simulink model "Simulink_Control_BlueROVtest6"  (R2022b)
settings: Solver=VariableStepAuto  StartTime=0.0  StopTime=20  RelTol=1e-3
model workspace (MAT data in the model file):
  Minv = Simulink.Parameter
  Minv.Value = [0.0780640124902  0  0  0  0  0; 0  0.0499750124938  0  0  0  0; 0  0  0.0457038391225  0  0  0; 0  0  0  3.57142857143  0  0; 0  0  0  0  3.57142857143  0; 0  0  0  0  0  3.57142857143]
  Minv.DataType = 'auto'
  Minv.Complexity = 'real'
  Minv.Dimensions = [6 6]
values from neighbouring files (symbols this model uses):
  B = 0    [Control_BlueROV_Modo_Deslizante.m]
  C = 1    [Control_BlueROV_Modo_Deslizante.m]
  epsilong = 1    [Control_BlueROV_Modo_Deslizante.m]
  Ix = 0.1836    [Control_BlueROV_Modo_Deslizante.m]
  Ixy = 0    [Control_BlueROV_Modo_Deslizante.m]
  Ixz = 0    [Control_BlueROV_Modo_Deslizante.m]
  Iy = 0.2181    [Control_BlueROV_Modo_Deslizante.m]
  Iyz = -0.0021    [Control_BlueROV_Modo_Deslizante.m]
  Iz = 0.1482    [Control_BlueROV_Modo_Deslizante.m]
  K = 5    [Control_BlueROV_Modo_Deslizante.m]
  Kp = -5.005    [Control_BlueROV_Modo_Deslizante.m]
  Kpdot = -0.8576    [Control_BlueROV_Modo_Deslizante.m]
  Kpp = -80.25    [Control_BlueROV_Modo_Deslizante.m]
  m = 10.7668    [Control_BlueROV_Modo_Deslizante.m]
  M = Mrb+Ma    [Control_BlueROV_Modo_Deslizante.m]
  Minv = inv(M)    [Control_BlueROV_Modo_Deslizante.m]
  Mq = -5.005    [Control_BlueROV_Modo_Deslizante.m]
  Mqdot = -1.1214    [Control_BlueROV_Modo_Deslizante.m]
  Mqq = -80.25    [Control_BlueROV_Modo_Deslizante.m]
  Nr = -0.004    [Control_BlueROV_Modo_Deslizante.m]
  Nrdot = -0.7399    [Control_BlueROV_Modo_Deslizante.m]
  Nrr = -0.2506    [Control_BlueROV_Modo_Deslizante.m]
  W = 0    [Control_BlueROV_Modo_Deslizante.m]
  xb = 0    [Control_BlueROV_Modo_Deslizante.m]
  xg = 0    [Control_BlueROV_Modo_Deslizante.m]
  Xu = -0.0048    [Control_BlueROV_Modo_Deslizante.m]
  Xudot = -4.9063    [Control_BlueROV_Modo_Deslizante.m]
  Xuu = -30.61    [Control_BlueROV_Modo_Deslizante.m]
  yb = 0    [Control_BlueROV_Modo_Deslizante.m]
  yg = 0    [Control_BlueROV_Modo_Deslizante.m]
  Yv = -0.2437    [Control_BlueROV_Modo_Deslizante.m]
  Yvdot = -9.9210    (= -9.921)    [Control_BlueROV_Modo_Deslizante.m]
  Yvv = -38.0036    [Control_BlueROV_Modo_Deslizante.m]
  zb = 0.02    [Control_BlueROV_Modo_Deslizante.m]
  zg = 0    [Control_BlueROV_Modo_Deslizante.m]
  Zw = -0.0094    [Control_BlueROV_Modo_Deslizante.m]
  Zwdot = -17.6159    [Control_BlueROV_Modo_Deslizante.m]
  Zww = -62.5364    [Control_BlueROV_Modo_Deslizante.m]
libraries: simulink x1
(part 1 of 3)
settings Model: Creator=andres lopez  LastModifiedBy=Administrator
settings SolverCC: ZeroCrossAlgorithm=Adaptive  AlgebraicLoopSolver=TrustRegion
settings DebuggingCC: IgnoredZcDiagnostic=none  UnconnectedInputMsg=warning  UnconnectedOutputMsg=warning  UnconnectedLineMsg=warning  SFMachineParentedDataDiag=warning
settings ModelReferenceCC: EnableRefExpFcnMdlSchedulingChecks=on
settings SFSimCC: CustomCodeUndefinedFunction=UseInterfaceOnly

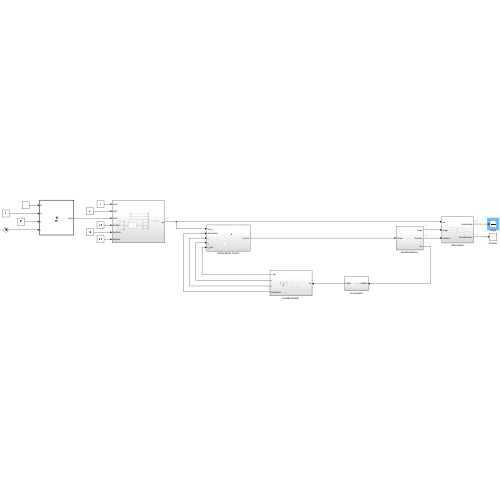
[thumbnail: Simulink's stored preview of the top-level diagram]
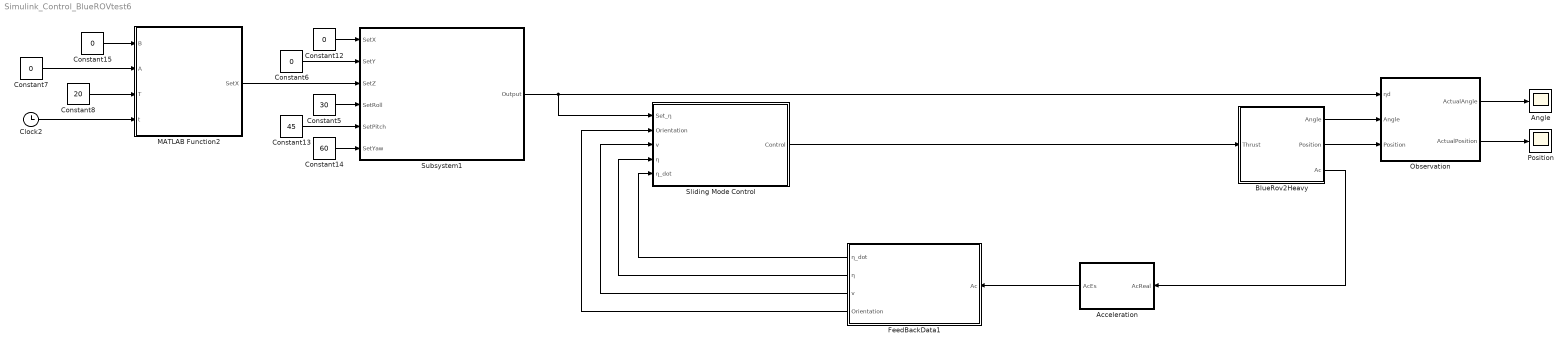
== system Simulink_Control_BlueROVtest6 ==
  Acceleration : Subsystem
  Angle : Scope
  BlueRov2Heavy : Subsystem
  Clock2 : Clock
  Constant{6..7,12,15} (4 alike) : Constant  Value=0
  Constant13 : Constant  Value=45
  Constant14 : Constant  Value=60
  Constant5 : Constant  Value=30
  Constant8 : Constant  Value=20
  FeedBackData1 : Subsystem
  MATLAB Function2 : MATLAB Function  TreatAsAtomicUnit=on
  Observation : Subsystem
  Position : Scope
  Sliding Mode Control : Subsystem
  Subsystem1 : Subsystem
  wires:
  Observation/1(ActualAngle) -> Angle/1
  BlueRov2Heavy/1(Angle) -> Observation/2(Angle)
  Observation/2(ActualPosition) -> Position/1
  Constant14/1 -> Subsystem1/6(SetYaw)
  Constant6/1 -> Subsystem1/2(SetY)
  Constant8/1 -> MATLAB Function2/3(T)
  Clock2/1 -> MATLAB Function2/4(t)
  Constant13/1 -> Subsystem1/5(SetPitch)
  Constant15/1 -> MATLAB Function2/1(B)
  Constant5/1 -> Subsystem1/4(SetRoll)
  Constant7/1 -> MATLAB Function2/2(A)
  Constant12/1 -> Subsystem1/1(SetX)
  MATLAB Function2/1(SetX) -> Subsystem1/3(SetZ)
  BlueRov2Heavy/2(Position) -> Observation/3(Position)
  Acceleration/1(AcEs) -> FeedBackData1/1(Ac)
  BlueRov2Heavy/3(Ac) -> Acceleration/1(AcReal)
  FeedBackData1/1(η_dot) -> Sliding Mode Control/5(η_dot)
  FeedBackData1/2(η) -> Sliding Mode Control/4(η)
  FeedBackData1/3(v) -> Sliding Mode Control/3(v)
  FeedBackData1/4(Orientation) -> Sliding Mode Control/2(Orientation)
  Subsystem1/1(Output) -> Observation/1(ηd), Sliding Mode Control/1(Set_η)
  Sliding Mode Control/1(Control) -> BlueRov2Heavy/1(Thrust)

== system Simulink_Control_BlueROVtest6/Acceleration ==
  AcReal : Inport
  Gain : Gain
  AcEs : Outport  VectorParamsAs1DForOutWhenUnconnected=off
  wires:
  Gain/1 -> AcEs/1
  AcReal/1 -> Gain/1

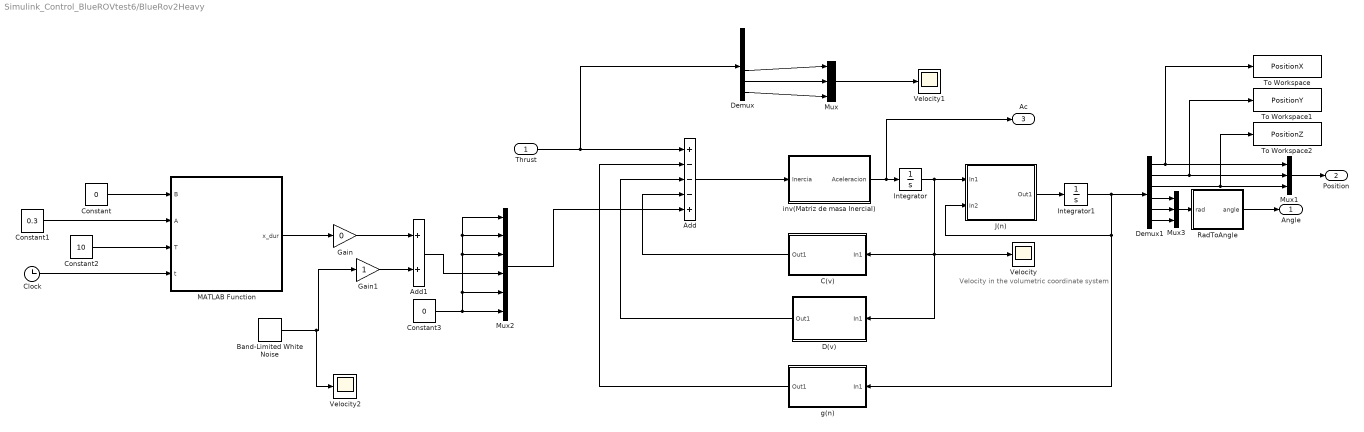
== system Simulink_Control_BlueROVtest6/BlueRov2Heavy ==
  note: Velocity in the volumetric coordinate system
  Thrust : Inport
  Add : Sum  Inputs=+---+
  Add1 : Sum
  Band-Limited White Noise : simulink/Sources/Band-Limited White Noise  Cov=[0.1]  Ts=0.1  seed=[23341]
  C(v) : Subsystem
  Clock : Clock
  Constant : Constant  Value=0
  Constant1 : Constant  Value=0.3
  Constant2 : Constant  Value=10
  Constant3 : Constant  Value=0
  D(v) : Subsystem
  Demux : Demux  Outputs=6
  Demux1 : Demux  Outputs=6
  Gain : Gain  Gain=0
  Gain1 : Gain
  Integrator : Integrator
  Integrator1 : Integrator
  J(n) : Subsystem
  MATLAB Function : MATLAB Function  TreatAsAtomicUnit=on
  Mux : Mux  Inputs=3
  Mux1 : Mux  Inputs=3
  Mux2 : Mux  Inputs=6
  Mux3 : Mux  Inputs=3
  RadToAngle : Subsystem
  To Workspace : ToWorkspace  VariableName=PositionX  SampleTime=-1
  To Workspace1 : ToWorkspace  VariableName=PositionY  SampleTime=-1
  To Workspace2 : ToWorkspace  VariableName=PositionZ  SampleTime=-1
  Velocity : Scope
  Velocity1 : Scope
  Velocity2 : Scope
  g(n) : Subsystem
  inv(Matriz de masa Inercial) : Subsystem
  Angle : Outport  VectorParamsAs1DForOutWhenUnconnected=off
  Position : Outport  Port=2  VectorParamsAs1DForOutWhenUnconnected=off
  Ac : Outport  Port=3  VectorParamsAs1DForOutWhenUnconnected=off
  wires:
  Thrust/1 -> Demux/1, Add/1
  Add/1 -> inv(Matriz de masa Inercial)/1(Inercia)
  J(n)/1(Out1) -> Integrator1/1
  inv(Matriz de masa Inercial)/1(Aceleracion) -> Ac/1, Integrator/1
  g(n)/1(Out1) -> Add/2
  Integrator1/1 -> g(n)/1(In1), J(n)/2(In2), Demux1/1
  Integrator/1 -> Velocity/1, D(v)/1(In1), C(v)/1(In1), J(n)/1(In1)
  C(v)/1(Out1) -> Add/4
  Demux1/2 -> To Workspace1/1, Mux1/2
  Demux1/3 -> To Workspace2/1, Mux1/3
  Demux1/1 -> To Workspace/1, Mux1/1
  Mux1/1 -> Position/1
  D(v)/1(Out1) -> Add/3
  Constant/1 -> MATLAB Function/1(B)
  Constant1/1 -> MATLAB Function/2(A)
  Constant2/1 -> MATLAB Function/3(T)
  Clock/1 -> MATLAB Function/4(t)
  Mux2/1 -> Add/5
  Constant3/1 -> Mux2/3, Mux2/2, Mux2/1, Mux2/5, Mux2/6
  MATLAB Function/1(x_dur) -> Gain/1
  Gain/1 -> Add1/1
  Gain1/1 -> Add1/2
  Mux3/1 -> RadToAngle/1(rad)
  Demux1/5 -> Mux3/2
  Demux1/4 -> Mux3/1
  Demux1/6 -> Mux3/3
  RadToAngle/1(angle) -> Angle/1
  Band-Limited White Noise/1 -> Velocity2/1, Gain1/1
  Demux/4 -> Mux/1
  Demux/5 -> Mux/2
  Demux/6 -> Mux/3
  Mux/1 -> Velocity1/1
  Add1/1 -> Mux2/4

== system Simulink_Control_BlueROVtest6/FeedBackData1 ==
  note: 输入：体坐标系中的线加速度与角加速度
  note: 输出1：世界坐标系中的位置与角度
  note: 输出4：世界坐标系中的机器人角度信息
  Ac : Inport
  Demux : Demux  Outputs=6
  Demux1 : Demux  Outputs=3
  Integrator : Integrator
  Integrator1 : Integrator
  J(n) : Subsystem
  Mux : Mux  Inputs=6
  Mux1 : Mux  Inputs=3
  η_dot : Outport
  η : Outport  Port=2  VectorParamsAs1DForOutWhenUnconnected=off
  v : Outport  Port=3
  Orientation : Outport  Port=4  VectorParamsAs1DForOutWhenUnconnected=off
  wires:
  Ac/1 -> Integrator/1
  Integrator/1 -> v/1, J(n)/1(In1)
  J(n)/1(Output) -> η_dot/1, Integrator1/1
  Integrator1/1 -> Demux/1
  Demux/1 -> Mux/1
  Demux/2 -> Mux/2
  Demux1/2 -> Mux/5
  Demux1/1 -> Mux/4
  Demux1/3 -> Mux/6
  Mux/1 -> η/1
  Demux/3 -> Mux/3
  Mux1/1 -> Orientation/1, J(n)/2(In2), Demux1/1
  Demux/4 -> Mux1/1
  Demux/5 -> Mux1/2
  Demux/6 -> Mux1/3

== system Simulink_Control_BlueROVtest6/Observation ==
  ηd : Inport
  Angle : Inport  Port=2
  Position : Inport  Port=3
  Demux : Demux  Outputs=2
  Mux : Mux  Inputs=2
  Mux1 : Mux  Inputs=2
  RadToAngle : Subsystem
  ActualAngle : Outport
  ActualPosition : Outport  Port=2
  wires:
  Demux/1 -> Mux/1
  Position/1 -> Mux/2
  Demux/2 -> RadToAngle/1(rad)
  Mux1/1 -> ActualAngle/1
  Mux/1 -> ActualPosition/1
  ηd/1 -> Demux/1
  RadToAngle/1(angle) -> Mux1/1
  Angle/1 -> Mux1/2

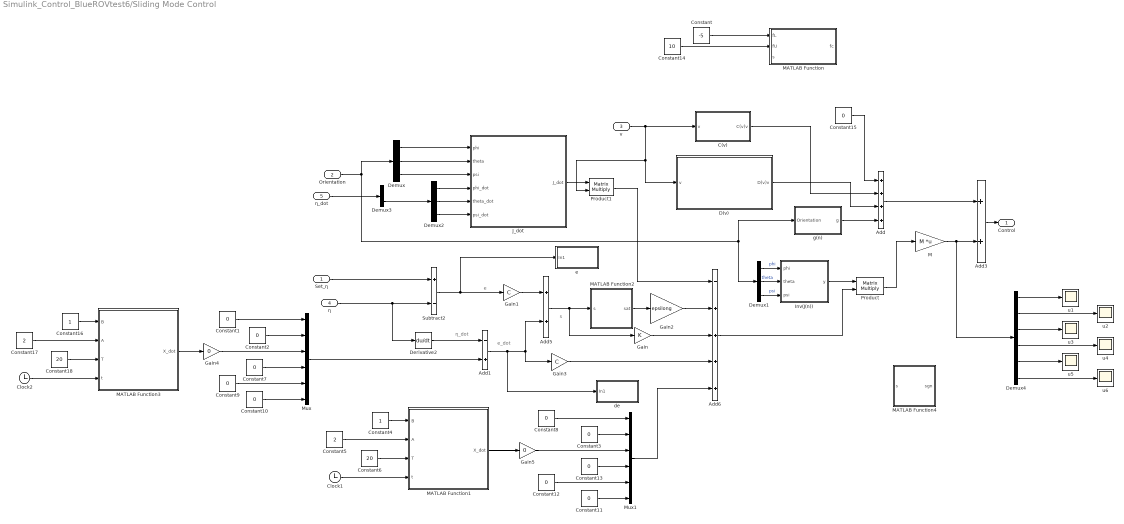
== system Simulink_Control_BlueROVtest6/Sliding Mode Control ==
  note: η_dot
  note: s
  note: e
  note: e_dot
  Set_η : Inport
  Orientation : Inport  Port=2
  v : Inport  Port=3
  η : Inport  Port=4
  η_dot : Inport  Port=5
  Add : Sum  Inputs=++++
  Add1 : Sum  Inputs=-+
  Add3 : Sum
  Add5 : Sum
  Add6 : Sum  Inputs=-++++
  C(v) : Subsystem
  Clock1 : Clock
  Clock2 : Clock
  Constant : Constant  Value=-5
  Constant{1..3,7..13,15} (11 alike) : Constant  Value=0
  Constant14 : Constant  Value=10
  Constant16 : Constant
  Constant17 : Constant  Value=2
  Constant18 : Constant  Value=20
  Constant4 : Constant
  Constant5 : Constant  Value=2
  Constant6 : Constant  Value=20
  D(v) : Subsystem
  Demux : Demux  Outputs=3
  Demux1 : Demux  Outputs=3
  Demux2 : Demux  Outputs=3
  Demux3 : Demux  Outputs=2
  Demux4 : Demux  Outputs=6
  Derivative2 : Derivative
  Gain : Gain  Gain=K
  Gain1 : Gain  Gain=C
  Gain2 : Gain  Gain=epsilong
  Gain3 : Gain  Gain=C
  Gain4 : Gain  Gain=0
  Gain5 : Gain  Gain=0
  Inv(J(n)) : MATLAB Function  TreatAsAtomicUnit=on
  J_dot : MATLAB Function  TreatAsAtomicUnit=on
  M : Gain  Gain=M  Multiplication=Matrix(K*u) (u vector)
  MATLAB Function : MATLAB Function  TreatAsAtomicUnit=on
  MATLAB Function1 : MATLAB Function  TreatAsAtomicUnit=on
  MATLAB Function2 : MATLAB Function  TreatAsAtomicUnit=on
  MATLAB Function3 : MATLAB Function  TreatAsAtomicUnit=on
  MATLAB Function4 : MATLAB Function  TreatAsAtomicUnit=on
  Mux : Mux  Inputs=6
  Mux1 : Mux  Inputs=6
  Product : Product  Multiplication=Matrix(*)
  Product1 : Product  Multiplication=Matrix(*)
  Subtract2 : Sum  Inputs=+-
  de : Subsystem
  e : Subsystem
  g(n) : Subsystem
  u{1..6} (6 alike) : Scope
  Control : Outport  VectorParamsAs1DForOutWhenUnconnected=off
  wires:
  Orientation/1 -> g(n)/1(Orientation), Demux1/1, Demux/1
  Demux1/1 -> Inv(J(n))/1(phi)  "phi"
  Demux1/3 -> Inv(J(n))/3(psi)  "psi"
  Inv(J(n))/1(y) -> Product/1
  Demux1/2 -> Inv(J(n))/2(theta)  "theta"
  Add3/1 -> Control/1
  M/1 -> Add3/2, Demux4/1
  Add/1 -> Add3/1
  η/1 -> Derivative2/1, Subtract2/2
  Set_η/1 -> Subtract2/1
  v/1 -> D(v)/1(v), Product1/2, C(v)/1(v)
  Add1/1 -> de/1(In1), Add5/2, Gain3/1
  Gain1/1 -> Add5/1
  Add5/1 -> MATLAB Function2/1(s), Gain/1
  Add6/1 -> Product/2
  Subtract2/1 -> e/1(In1), Gain1/1
  Product/1 -> M/1
  Demux/1 -> J_dot/1(phi)
  Demux/2 -> J_dot/2(theta)
  Demux/3 -> J_dot/3(psi)
  Demux2/1 -> J_dot/4(phi_dot)
  Demux2/2 -> J_dot/5(theta_dot)
  Demux2/3 -> J_dot/6(psi_dot)
  Gain/1 -> Add6/3
  Product1/1 -> Add6/1
  J_dot/1(J_dot) -> Product1/1
  Gain3/1 -> Add6/4
  Demux3/2 -> Demux2/1
  η_dot/1 -> Demux3/1
  Derivative2/1 -> Add1/1
  Constant7/1 -> Mux/4
  Constant10/1 -> Mux/6
  Constant9/1 -> Mux/5
  Constant11/1 -> Mux1/6
  Constant12/1 -> Mux1/5
  Constant13/1 -> Mux1/4
  Mux/1 -> Add1/2
  Mux1/1 -> Add6/5
  Constant18/1 -> MATLAB Function3/3(T)
  Constant16/1 -> MATLAB Function3/1(B)
  Constant17/1 -> MATLAB Function3/2(A)
  Clock2/1 -> MATLAB Function3/4(t)
  MATLAB Function1/1(X_dot) -> Gain5/1
  Gain2/1 -> Add6/2
  MATLAB Function2/1(sat) -> Gain2/1
  MATLAB Function3/1(X_dot) -> Gain4/1
  Constant2/1 -> Mux/2
  Constant3/1 -> Mux1/2
  Constant4/1 -> MATLAB Function1/1(B)
  Constant5/1 -> MATLAB Function1/2(A)
  Clock1/1 -> MATLAB Function1/4(t)
  Constant6/1 -> MATLAB Function1/3(T)
  Constant1/1 -> Mux/1
  Constant8/1 -> Mux1/1
  Demux4/1 -> u1/1
  Demux4/2 -> u2/1
  Demux4/3 -> u3/1
  Demux4/4 -> u4/1
  Demux4/5 -> u5/1
  Demux4/6 -> u6/1
  Constant14/1 -> MATLAB Function/2(fU)
  Constant/1 -> MATLAB Function/1(fL)
  g(n)/1(g) -> Add/4
  D(v)/1(D(v)v) -> Add/3
  C(v)/1(C(v)v) -> Add/2
  Constant15/1 -> Add/1
  Gain4/1 -> Mux/3
  Gain5/1 -> Mux1/3

== system Simulink_Control_BlueROVtest6/Subsystem1 ==
  SetX : Inport
  SetY : Inport  Port=2
  SetZ : Inport  Port=3
  SetRoll : Inport  Port=4
  SetPitch : Inport  Port=5
  SetYaw : Inport  Port=6
  AngleToRad : Subsystem
  Demux : Demux  Outputs=3
  Mux : Mux  Inputs=3
  Mux1 : Mux  Inputs=6
  Output : Outport
  wires:
  SetY/1 -> Mux1/2
  Mux1/1 -> Output/1  "ηd"
  SetZ/1 -> Mux1/3
  SetX/1 -> Mux1/1
  Demux/1 -> Mux1/4
  Demux/2 -> Mux1/5
  Demux/3 -> Mux1/6
  AngleToRad/1(Rad) -> Demux/1
  Mux/1 -> AngleToRad/1(Angle)
  SetRoll/1 -> Mux/1
  SetPitch/1 -> Mux/2
  SetYaw/1 -> Mux/3

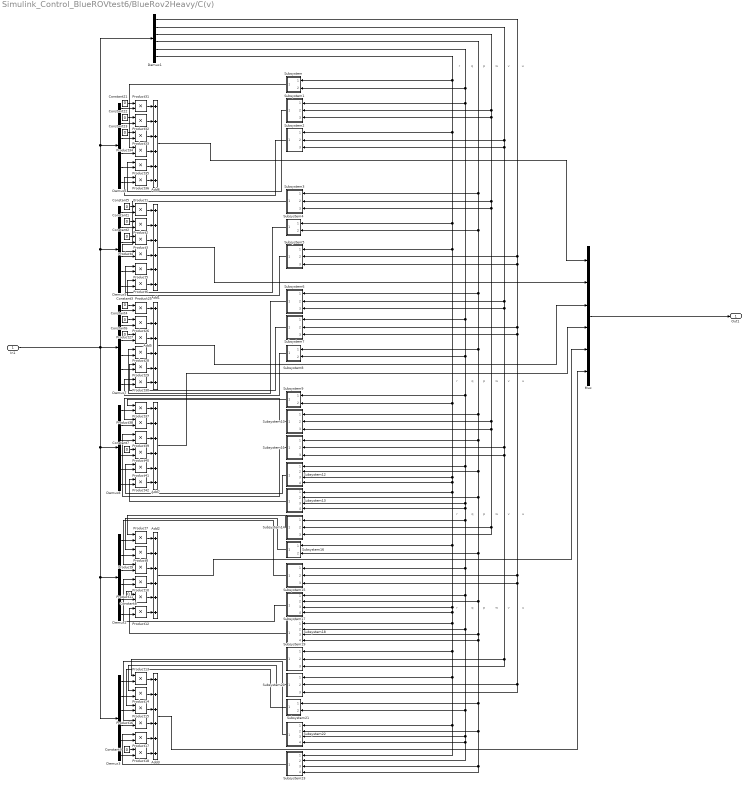
== system Simulink_Control_BlueROVtest6/BlueRov2Heavy/C(v) ==
  note: u
  note: v
  note: w
  note: p
  note: q
  note: r
  note: v
  note: p
  note: u
  note: w
  note: q
  note: r
  note: v
  note: r
  note: w
  note: u
  note: q
  note: p
  note: v
  note: r
  note: w
  note: u
  note: q
  note: p
  In1 : Inport
  Add{1..3,5..7} (6 alike) : Sum  Inputs=++++++
  Constant{1..9,21..23} (12 alike) : Constant  Value=0
  Demux{1..3,5..8} (7 alike) : Demux  Outputs=6
  Mux : Mux  Inputs=6
  Product{1..18,25..42} (36 alike) : Product
  Subsystem : Subsystem
  Subsystem1 : Subsystem
  Subsystem10 : Subsystem
  Subsystem11 : Subsystem
  Subsystem12 : Subsystem
  Subsystem13 : Subsystem
  Subsystem14 : Subsystem
  Subsystem15 : Subsystem
  Subsystem16 : Subsystem
  Subsystem17 : Subsystem
  Subsystem18 : Subsystem
  Subsystem19 : Subsystem
  Subsystem2 : Subsystem
  Subsystem20 : Subsystem
  Subsystem21 : Subsystem
  Subsystem22 : Subsystem
  Subsystem23 : Subsystem
  Subsystem3 : Subsystem
  Subsystem4 : Subsystem
  Subsystem5 : Subsystem
  Subsystem6 : Subsystem
  Subsystem7 : Subsystem
  Subsystem8 : Subsystem
  Subsystem9 : Subsystem
  Out1 : Outport  VectorParamsAs1DForOutWhenUnconnected=off
  wires:
  In1/1 -> Demux5/1, Demux6/1, Demux1/1, Demux7/1, Demux8/1, Demux3/1, Demux2/1
  Product39/1 -> Add7/3
  Demux8/2 -> Product38/2
  Product36/1 -> Add6/6
  Product31/1 -> Add6/1
  Product35/1 -> Add6/5
  Demux6/2 -> Product32/2
  Demux6/4 -> Product34/2
  Demux6/5 -> Product35/2
  Product33/1 -> Add6/3
  Demux6/3 -> Product33/2
  Product5/1 -> Add1/5
  Demux5/2 -> Product2/2
  Product32/1 -> Add6/2
  Product41/1 -> Add7/5
  Product34/1 -> Add6/4
  Product2/1 -> Add1/2
  Demux8/5 -> Product41/2
  Product1/1 -> Add1/1
  Product18/1 -> Add3/6
  Product3/1 -> Add1/3
  Demux8/3 -> Product39/2
  Product8/1 -> Add2/2
  Demux2/6 -> Product12/2
  Product4/1 -> Add1/4
  Product37/1 -> Add7/1
  Demux5/1 -> Product1/2
  Demux8/6 -> Product42/2
  Demux5/4 -> Product4/2
  Demux5/5 -> Product5/2
  Product17/1 -> Add3/5
  Demux5/3 -> Product3/2
  Demux6/1 -> Product31/2
  Product13/1 -> Add3/1
  Product14/1 -> Add3/2
  Product40/1 -> Add7/4
  Product15/1 -> Add3/3
  Demux8/4 -> Product40/2
  Demux7/2 -> Product26/2
  Product42/1 -> Add7/6
  Product12/1 -> Add2/6
  Product26/1 -> Add5/2
  Product6/1 -> Add1/6
  Demux6/6 -> Product36/2
  Demux5/6 -> Product6/2
  Product29/1 -> Add5/5
  Product28/1 -> Add5/4
  Demux7/3 -> Product27/2
  Product16/1 -> Add3/4
  Product10/1 -> Add2/4
  Demux7/5 -> Product29/2
  Product9/1 -> Add2/3
  Product38/1 -> Add7/2
  Demux2/4 -> Product10/2
  Demux2/2 -> Product8/2
  Demux8/1 -> Product37/2
  Demux2/5 -> Product11/2
  Product7/1 -> Add2/1
  Product11/1 -> Add2/5
  Mux/1 -> Out1/1
  Demux7/4 -> Product28/2
  Demux2/1 -> Product7/2
  Demux7/6 -> Product30/2
  Product25/1 -> Add5/1
  Product27/1 -> Add5/3
  Product30/1 -> Add5/6
  Demux7/1 -> Product25/2
  Demux2/3 -> Product9/2
  Constant21/1 -> Product31/1
  Constant22/1 -> Product32/1
  Constant23/1 -> Product33/1
  Demux3/6 -> Product18/2
  Demux3/5 -> Product17/2
  Demux3/4 -> Product16/2
  Demux3/3 -> Product15/2
  Demux3/2 -> Product14/2
  Demux3/1 -> Product13/2
  Constant5/1 -> Product1/1
  Constant1/1 -> Product2/1
  Constant2/1 -> Product3/1
  Constant3/1 -> Product25/1
  Constant4/1 -> Product26/1
  Constant6/1 -> Product27/1
  Constant7/1 -> Product40/1
  Constant8/1 -> Product11/1
  Constant9/1 -> Product18/1
  Demux1/1 -> Subsystem5/2(In2), Subsystem15/2(In2), Subsystem15/3(In3), Subsystem20/2(In2), Subsystem20/3(In3), Subsystem7/3(In3), Subsystem7/2(In2), Subsystem5/3(In3)
  Demux1/2 -> Subsystem11/3(In3), Subsystem19/2(In2), Subsystem19/3(In3), Subsystem11/2(In2), Subsystem6/3(In3), Subsystem6/2(In2), Subsystem2/3(In3), Subsystem2/2(In2)
  Demux1/3 -> Subsystem3/2(In2), Subsystem3/3(In3), Subsystem10/2(In2), Subsystem10/3(In3), Subsystem14/2(In2), Subsystem14/3(In3), Subsystem1/3(In3), Subsystem1/2(In2)
  Subsystem/1(Out1) -> Product34/1
  Subsystem1/1(Out1) -> Product35/1
  Subsystem2/1(Out1) -> Product36/1
  Add6/1 -> Mux/1
  Subsystem3/1(Out1) -> Product4/1
  Subsystem4/1(Out1) -> Product5/1
  Subsystem5/1(Out1) -> Product6/1
  Add1/1 -> Mux/2
  Subsystem6/1(Out1) -> Product28/1
  Subsystem7/1(Out1) -> Product29/1
  Subsystem8/1(Out1) -> Product30/1
  Add5/1 -> Mux/3
  Subsystem9/1(Out1) -> Product37/1
  Subsystem10/1(Out1) -> Product38/1
  Subsystem11/1(Out1) -> Product39/1
  Subsystem12/1(Out1) -> Product41/1
  Subsystem13/1(Out1) -> Product42/1
  Add7/1 -> Mux/4
  Subsystem14/1(Out1) -> Product7/1
  Demux1/4 -> Subsystem3/1(In1), Subsystem4/2(In2), Subsystem8/1(In1), Subsystem10/1(In1), Subsystem11/1(In1), Subsystem12/2(In2), Subsystem13/2(In2), Subsystem16/2(In2), Subsystem17/2(In2), Subsystem18/3(In3), Subsystem18/4(In4), Subsystem21/1(In1), Subsystem22/2(In2), Subsystem23/3(In3), Subsystem23/4(In4), Subsystem6/1(In1)
  Subsystem16/1(Out1) -> Product8/1
  Subsystem15/1(Out1) -> Product9/1
  Demux1/6 -> Subsystem4/1(In1), Subsystem5/1(In1), Subsystem12/4(In4), Subsystem13/1(In1), Subsystem16/1(In1), Subsystem17/4(In4), Subsystem18/1(In1), Subsystem19/1(In1), Subsystem20/1(In1), Subsystem22/1(In1), Subsystem23/1(In1), Subsystem17/3(In3), Subsystem12/3(In3), Subsystem9/2(In2), Subsystem2/1(In1), Subsystem/1(In1)
  Subsystem17/1(Out1) -> Product10/1
  Subsystem18/1(Out1) -> Product12/1
  Subsystem19/1(Out1) -> Product13/1
  Add2/1 -> Mux/5
  Subsystem20/1(Out1) -> Product14/1
  Subsystem21/1(Out1) -> Product15/1
  Demux1/5 -> Subsystem12/1(In1), Subsystem13/3(In3), Subsystem13/4(In4), Subsystem15/1(In1), Subsystem17/1(In1), Subsystem18/2(In2), Subsystem21/2(In2), Subsystem22/4(In4), Subsystem23/2(In2), Subsystem22/3(In3), Subsystem14/1(In1), Subsystem9/1(In1), Subsystem8/2(In2), Subsystem7/1(In1), Subsystem1/1(In1), Subsystem/2(In2)
  Subsystem22/1(Out1) -> Product16/1
  Subsystem23/1(Out1) -> Product17/1
  Add3/1 -> Mux/6

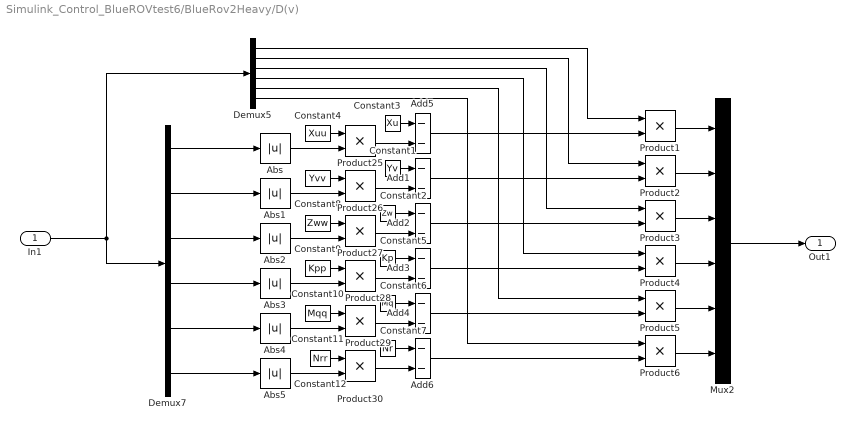
== system Simulink_Control_BlueROVtest6/BlueRov2Heavy/D(v) ==
  In1 : Inport
  Abs{,1..5} (6 alike) : Abs  SaturateOnIntegerOverflow=off
  Add{1..6} (6 alike) : Sum  Inputs=--
  Constant1 : Constant  Value=Yv
  Constant10 : Constant  Value=Kpp
  Constant11 : Constant  Value=Mqq
  Constant12 : Constant  Value=Nrr
  Constant2 : Constant  Value=Zw
  Constant3 : Constant  Value=Xu
  Constant4 : Constant  Value=Xuu
  Constant5 : Constant  Value=Kp
  Constant6 : Constant  Value=Mq
  Constant7 : Constant  Value=Nr
  Constant8 : Constant  Value=Yvv
  Constant9 : Constant  Value=Zww
  Demux5 : Demux  Outputs=6
  Demux7 : Demux  Outputs=6
  Mux2 : Mux  Inputs=6
  Product{1..6,25..30} (12 alike) : Product
  Out1 : Outport
  wires:
  Demux5/5 -> Product5/1
  Demux7/3 -> Abs2/1
  Abs/1 -> Product25/2
  Demux7/5 -> Abs4/1
  Constant9/1 -> Product27/1
  Constant6/1 -> Add4/1
  Mux2/1 -> Out1/1
  Constant1/1 -> Add1/1
  Product5/1 -> Mux2/5
  Abs1/1 -> Product26/2
  Product4/1 -> Mux2/4
  Constant2/1 -> Add2/1
  Demux7/4 -> Abs3/1
  Demux7/6 -> Abs5/1
  Constant12/1 -> Product30/1
  In1/1 -> Demux5/1, Demux7/1
  Product1/1 -> Mux2/1
  Demux7/1 -> Abs/1
  Product29/1 -> Add4/2
  Add3/1 -> Product4/2
  Constant10/1 -> Product28/1
  Add1/1 -> Product2/2
  Demux7/2 -> Abs1/1
  Product26/1 -> Add1/2
  Demux5/2 -> Product2/1
  Add4/1 -> Product5/2
  Demux5/4 -> Product4/1
  Abs5/1 -> Product30/2
  Product3/1 -> Mux2/3
  Product6/1 -> Mux2/6
  Abs3/1 -> Product28/2
  Constant4/1 -> Product25/1
  Constant11/1 -> Product29/1
  Product28/1 -> Add3/2
  Product25/1 -> Add5/2
  Abs2/1 -> Product27/2
  Constant7/1 -> Add6/1
  Demux5/6 -> Product6/1
  Product27/1 -> Add2/2
  Add2/1 -> Product3/2
  Constant3/1 -> Add5/1
  Product30/1 -> Add6/2
  Abs4/1 -> Product29/2
  Constant5/1 -> Add3/1
  Product2/1 -> Mux2/2
  Demux5/1 -> Product1/1
  Constant8/1 -> Product26/1
  Add5/1 -> Product1/2
  Demux5/3 -> Product3/1
  Add6/1 -> Product6/2

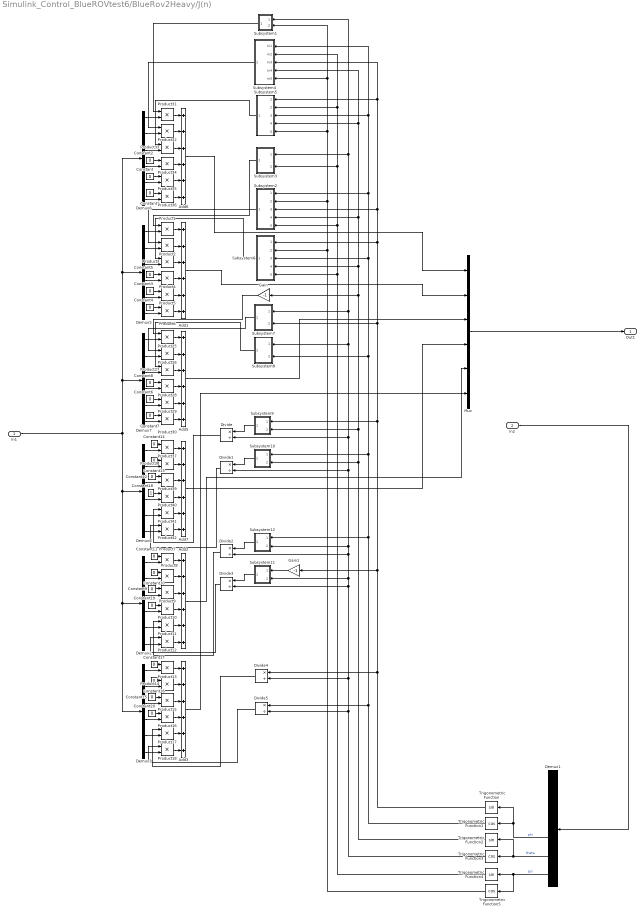
== system Simulink_Control_BlueROVtest6/BlueRov2Heavy/J(n) ==
  In1 : Inport
  In2 : Inport  Port=2
  Add{1..3,5..7} (6 alike) : Sum  Inputs=++++++
  Constant{,1..17,19..20} (20 alike) : Constant  Value=0
  Constant18 : Constant
  Demux{1..3,5..8} (7 alike) : Demux  Outputs=6
  Divide{,1..5} (6 alike) : Product  Inputs=*/
  Gain : Gain  Gain=-1
  Gain1 : Gain  Gain=-1
  Mux : Mux  Inputs=6
  Product{1..18,25..42} (36 alike) : Product
  Subsystem1 : Subsystem
  Subsystem10 : Subsystem
  Subsystem11 : Subsystem
  Subsystem12 : Subsystem
  Subsystem2 : Subsystem
  Subsystem3 : Subsystem
  Subsystem4 : Subsystem
  Subsystem5 : Subsystem
  Subsystem6 : Subsystem
  Subsystem7 : Subsystem
  Subsystem8 : Subsystem
  Subsystem9 : Subsystem
  Trigonometric Function : Trigonometry
  Trigonometric Function1 : Trigonometry  Operator=cos
  Trigonometric Function2 : Trigonometry
  Trigonometric Function3 : Trigonometry  Operator=cos
  Trigonometric Function4 : Trigonometry
  Trigonometric Function5 : Trigonometry  Operator=cos
  Out1 : Outport  VectorParamsAs1DForOutWhenUnconnected=off
  wires:
  Divide5/1 -> Product18/1
  Divide3/1 -> Product12/1
  Subsystem1/1(Out1) -> Product31/1
  Constant12/1 -> Product39/1
  Subsystem5/1(Out1) -> Product33/1
  Constant13/1 -> Product38/1
  Subsystem10/1(Out1) -> Divide1/1
  Divide1/1 -> Product42/1
  Demux7/3 -> Product27/2
  Product28/1 -> Add5/4
  Product29/1 -> Add5/5
  Product25/1 -> Add5/1
  Product30/1 -> Add5/6
  Demux7/6 -> Product30/2
  Constant8/1 -> Product28/1
  Demux7/1 -> Product25/2
  Demux7/4 -> Product28/2
  Product27/1 -> Add5/3
  Constant6/1 -> Product29/1
  Product11/1 -> Add2/5
  Demux2/3 -> Product9/2
  Product7/1 -> Add2/1
  Demux2/1 -> Product7/2
  Demux2/5 -> Product11/2
  Demux2/4 -> Product10/2
  Product9/1 -> Add2/3
  Demux2/2 -> Product8/2
  Constant10/1 -> Product8/1
  Trigonometric Function3/1 -> Divide5/2, Divide4/2, Divide3/2, Subsystem11/2(In2), Divide2/2, Subsystem12/2(In2), Divide1/2, Divide/2, Subsystem8/1(In1), Subsystem7/1(In1), Subsystem3/1(In1), Subsystem1/1(In1)
  Demux8/2 -> Product38/2
  Product39/1 -> Add7/3
  Product38/1 -> Add7/2
  In1/1 -> Demux5/1, Demux6/1, Demux7/1, Demux8/1, Demux3/1, Demux2/1
  Subsystem9/1(Out1) -> Divide/1
  Add2/1 -> Mux/5
  Subsystem11/1(Out1) -> Divide3/1
  Product10/1 -> Add2/4
  Subsystem12/1(Out1) -> Divide2/1
  Constant19/1 -> Product10/1
  Trigonometric Function1/1 -> Divide5/1, Subsystem10/1(In1), Subsystem8/2(In2), Subsystem6/3(In3), Subsystem2/1(In1), Subsystem5/3(In3), Subsystem4/1(In1), Subsystem12/1(In1)
  Add1/1 -> Mux/2
  Mux/1 -> Out1/1
  Add6/1 -> Mux/1
  Add3/1 -> Mux/6
  Product12/1 -> Add2/6
  Add7/1 -> Mux/4
  Divide4/1 -> Product17/1
  Add5/1 -> Mux/3
  Product26/1 -> Add5/2
  Constant7/1 -> Product30/1
  Trigonometric Function/1 -> Divide4/1, Gain1/1, Subsystem9/1(In1), Subsystem7/2(In2), Subsystem6/1(In1), Subsystem2/3(In3), Subsystem5/1(In1), Subsystem4/3(In3)
  Constant14/1 -> Product37/1
  Gain/1 -> Product25/1
  Trigonometric Function5/1 -> Subsystem6/2(In2), Subsystem5/5(In5), Subsystem4/5(In5), Subsystem1/2(In2), Subsystem2/2(In2)
  Subsystem8/1(Out1) -> Product27/1
  Subsystem3/1(Out1) -> Product1/1
  Subsystem6/1(Out1) -> Product3/1
  Demux7/2 -> Product26/2
  Constant20/1 -> Product16/1
  Subsystem7/1(Out1) -> Product26/1
  Demux7/5 -> Product29/2
  Constant15/1 -> Product15/1
  Constant16/1 -> Product14/1
  Demux3/2 -> Product14/2
  Product15/1 -> Add3/3
  Constant17/1 -> Product13/1
  Product14/1 -> Add3/2
  Constant11/1 -> Product7/1
  Trigonometric Function4/1 -> Subsystem6/5(In5), Subsystem2/5(In5), Subsystem3/2(In2), Subsystem5/2(In2), Subsystem4/2(In2)
  Subsystem4/1(Out1) -> Product32/1
  Product13/1 -> Add3/1
  Product16/1 -> Add3/4
  Demux3/1 -> Product13/2
  Demux3/4 -> Product16/2
  Demux3/3 -> Product15/2
  Trigonometric Function2/1 -> Subsystem10/2(In2), Subsystem9/2(In2), Gain/1, Subsystem6/4(In4), Subsystem2/4(In4), Subsystem5/4(In4), Subsystem4/4(In4)
  Constant1/1 -> Product36/1
  Product17/1 -> Add3/5
  Demux5/3 -> Product3/2
  Product6/1 -> Add1/6
  Demux5/5 -> Product5/2
  Demux5/4 -> Product4/2
  Demux5/1 -> Product1/2
  Demux1/4 -> Trigonometric Function/1, Trigonometric Function1/1  "phi"
  Constant4/1 -> Product6/1
  Constant2/1 -> Product34/1
  Constant/1 -> Product35/1
  Demux8/6 -> Product42/2
  Demux3/5 -> Product17/2
  Product4/1 -> Add1/4
  Constant18/1 -> Product40/1
  Product37/1 -> Add7/1
  Demux2/6 -> Product12/2
  Demux8/4 -> Product40/2
  Gain1/1 -> Subsystem11/1(In1)
  Product42/1 -> Add7/6
  Constant3/1 -> Product5/1
  Product8/1 -> Add2/2
  Demux8/5 -> Product41/2
  Product1/1 -> Add1/1
  Demux8/3 -> Product39/2
  Product3/1 -> Add1/3
  Divide2/1 -> Product11/1
  Product18/1 -> Add3/6
  Demux1/6 -> Trigonometric Function5/1, Trigonometric Function4/1  "psi"
  Constant5/1 -> Product4/1
  Demux5/2 -> Product2/2
  Divide/1 -> Product41/1
  Product32/1 -> Add6/2
  Product2/1 -> Add1/2
  Product34/1 -> Add6/4
  Demux6/1 -> Product31/2
  Demux6/6 -> Product36/2
  Product41/1 -> Add7/5
  Demux6/5 -> Product35/2
  Product5/1 -> Add1/5
  Constant9/1 -> Product9/1
  Demux3/6 -> Product18/2
  Product33/1 -> Add6/3
  Demux1/5 -> Trigonometric Function2/1, Trigonometric Function3/1  "theta"
  Demux6/4 -> Product34/2
  Demux6/3 -> Product33/2
  Demux5/6 -> Product6/2
  Product36/1 -> Add6/6
  Demux6/2 -> Product32/2
  Subsystem2/1(Out1) -> Product2/1
  Product40/1 -> Add7/4
  Demux8/1 -> Product37/2
  Product31/1 -> Add6/1
  Product35/1 -> Add6/5
  In2/1 -> Demux1/1

== system Simulink_Control_BlueROVtest6/BlueRov2Heavy/RadToAngle ==
  rad : Inport
  Constant6 : Constant  Value=180
  Constant7 : Constant  Value=3.141592657
  Divide1 : Product  Inputs=*/*
  angle : Outport
  wires:
  Constant6/1 -> Divide1/3
  rad/1 -> Divide1/1
  Divide1/1 -> angle/1
  Constant7/1 -> Divide1/2

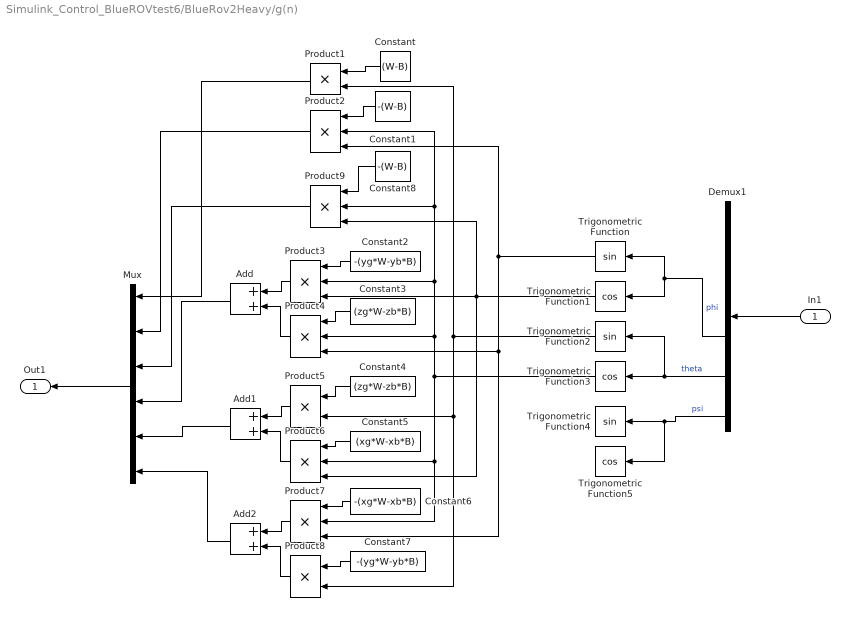
== system Simulink_Control_BlueROVtest6/BlueRov2Heavy/g(n) ==
  In1 : Inport
  Add : Sum
  Add1 : Sum
  Add2 : Sum
  Constant : Constant  Value=(W-B)
  Constant1 : Constant  Value=-(W-B)
  Constant2 : Constant  Value=-(yg*W-yb*B)
  Constant3 : Constant  Value=(zg*W-zb*B)
  Constant4 : Constant  Value=(zg*W-zb*B)
  Constant5 : Constant  Value=(xg*W-xb*B)
  Constant6 : Constant  Value=-(xg*W-xb*B)
  Constant7 : Constant  Value=-(yg*W-yb*B)
  Constant8 : Constant  Value=-(W-B)
  Demux1 : Demux  Outputs=6
  Mux : Mux  Inputs=6
  Product1 : Product
  Product{2..4,6..7,9} (6 alike) : Product  Inputs=3
  Product5 : Product
  Product8 : Product
  Trigonometric Function : Trigonometry
  Trigonometric Function1 : Trigonometry  Operator=cos
  Trigonometric Function2 : Trigonometry
  Trigonometric Function3 : Trigonometry  Operator=cos
  Trigonometric Function4 : Trigonometry
  Trigonometric Function5 : Trigonometry  Operator=cos
  Out1 : Outport  VectorParamsAs1DForOutWhenUnconnected=off
  wires:
  Demux1/6 -> Trigonometric Function5/1, Trigonometric Function4/1  "psi"
  Demux1/4 -> Trigonometric Function/1, Trigonometric Function1/1  "phi"
  Demux1/5 -> Trigonometric Function2/1, Trigonometric Function3/1  "theta"
  In1/1 -> Demux1/1
  Mux/1 -> Out1/1
  Product1/1 -> Mux/1
  Constant/1 -> Product1/1
  Trigonometric Function2/1 -> Product8/2, Product5/2, Product1/2
  Constant1/1 -> Product2/1
  Trigonometric Function/1 -> Product7/3, Product4/3, Product2/3
  Product2/1 -> Mux/2
  Product7/1 -> Add2/1
  Product8/1 -> Add2/2
  Product6/1 -> Add1/2
  Constant5/1 -> Product6/1
  Constant2/1 -> Product3/1
  Constant4/1 -> Product5/1
  Product4/1 -> Add/2
  Constant3/1 -> Product4/1
  Product3/1 -> Add/1
  Product5/1 -> Add1/1
  Constant7/1 -> Product8/1
  Constant8/1 -> Product9/1
  Product9/1 -> Mux/3
  Add/1 -> Mux/4
  Add1/1 -> Mux/5
  Constant6/1 -> Product7/1
  Add2/1 -> Mux/6
  Trigonometric Function1/1 -> Product6/3, Product3/3, Product9/3
  Trigonometric Function3/1 -> Product7/2, Product6/2, Product4/2, Product3/2, Product2/2, Product9/2

== system Simulink_Control_BlueROVtest6/BlueRov2Heavy/inv(Matriz de masa Inercial) ==
  note: 输出：体坐标系中的线加速度与角加速度
  Inercia : Inport
  INVM : Gain  Gain=Minv  Multiplication=Matrix(K*u) (u vector)
  Aceleracion : Outport  VectorParamsAs1DForOutWhenUnconnected=off
  wires:
  INVM/1 -> Aceleracion/1
  Inercia/1 -> INVM/1

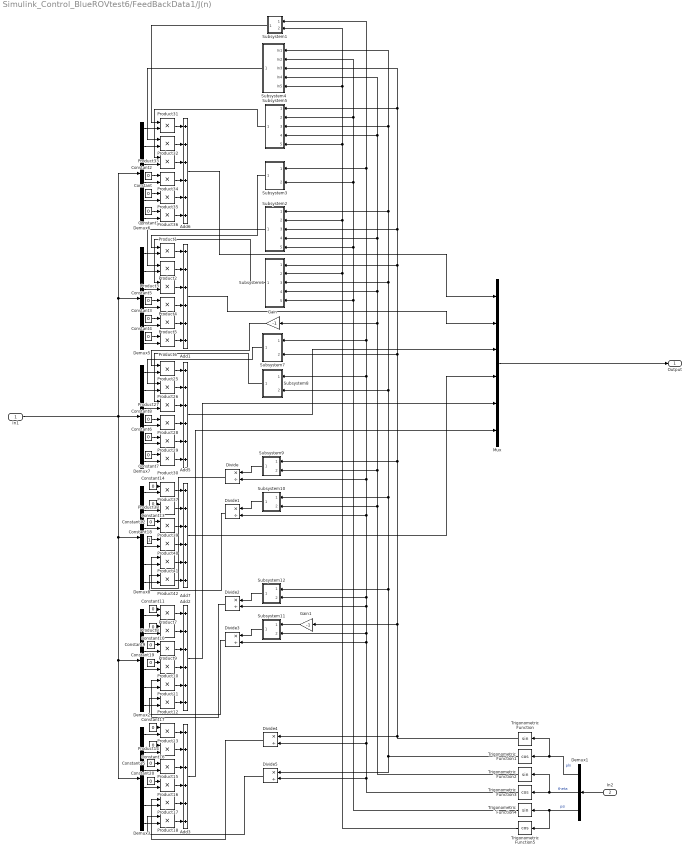
== system Simulink_Control_BlueROVtest6/FeedBackData1/J(n) ==
  In1 : Inport
  In2 : Inport  Port=2
  Add{1..3,5..7} (6 alike) : Sum  Inputs=++++++
  Constant{,1..17,19..20} (20 alike) : Constant  Value=0
  Constant18 : Constant
  Demux1 : Demux  Outputs=3
  Demux{2..3,5..8} (6 alike) : Demux  Outputs=6
  Divide{,1..5} (6 alike) : Product  Inputs=*/
  Gain : Gain  Gain=-1
  Gain1 : Gain  Gain=-1
  Mux : Mux  Inputs=6
  Product{1..18,25..42} (36 alike) : Product
  Subsystem1 : Subsystem
  Subsystem10 : Subsystem
  Subsystem11 : Subsystem
  Subsystem12 : Subsystem
  Subsystem2 : Subsystem
  Subsystem3 : Subsystem
  Subsystem4 : Subsystem
  Subsystem5 : Subsystem
  Subsystem6 : Subsystem
  Subsystem7 : Subsystem
  Subsystem8 : Subsystem
  Subsystem9 : Subsystem
  Trigonometric Function : Trigonometry
  Trigonometric Function1 : Trigonometry  Operator=cos
  Trigonometric Function2 : Trigonometry
  Trigonometric Function3 : Trigonometry  Operator=cos
  Trigonometric Function4 : Trigonometry
  Trigonometric Function5 : Trigonometry  Operator=cos
  Output : Outport  VectorParamsAs1DForOutWhenUnconnected=off
  wires:
  Divide5/1 -> Product18/1
  Divide3/1 -> Product12/1
  Subsystem1/1(Out1) -> Product31/1
  Constant12/1 -> Product39/1
  Subsystem5/1(Out1) -> Product33/1
  Constant13/1 -> Product38/1
  Subsystem10/1(Out1) -> Divide1/1
  Divide1/1 -> Product42/1
  Demux7/3 -> Product27/2
  Product28/1 -> Add5/4
  Product29/1 -> Add5/5
  Product25/1 -> Add5/1
  Product30/1 -> Add5/6
  Demux7/6 -> Product30/2
  Constant8/1 -> Product28/1
  Demux7/1 -> Product25/2
  Demux7/4 -> Product28/2
  Product27/1 -> Add5/3
  Constant6/1 -> Product29/1
  Product11/1 -> Add2/5
  Demux2/3 -> Product9/2
  Product7/1 -> Add2/1
  Demux2/1 -> Product7/2
  Demux2/5 -> Product11/2
  Demux2/4 -> Product10/2
  Product9/1 -> Add2/3
  Demux2/2 -> Product8/2
  Constant10/1 -> Product8/1
  Trigonometric Function3/1 -> Divide5/2, Divide4/2, Divide3/2, Subsystem11/2(In2), Divide2/2, Subsystem12/2(In2), Divide1/2, Divide/2, Subsystem8/1(In1), Subsystem7/1(In1), Subsystem3/1(In1), Subsystem1/1(In1)
  Demux8/2 -> Product38/2
  Product39/1 -> Add7/3
  Product38/1 -> Add7/2
  In1/1 -> Demux5/1, Demux6/1, Demux7/1, Demux8/1, Demux3/1, Demux2/1
  Subsystem9/1(Out1) -> Divide/1
  Add2/1 -> Mux/5
  Subsystem11/1(Out1) -> Divide3/1
  Product10/1 -> Add2/4
  Subsystem12/1(Out1) -> Divide2/1
  Constant19/1 -> Product10/1
  Trigonometric Function1/1 -> Divide5/1, Subsystem10/1(In1), Subsystem8/2(In2), Subsystem6/3(In3), Subsystem2/1(In1), Subsystem5/3(In3), Subsystem4/1(In1), Subsystem12/1(In1)
  Add1/1 -> Mux/2
  Mux/1 -> Output/1
  Add6/1 -> Mux/1
  Add3/1 -> Mux/6
  Product12/1 -> Add2/6
  Add7/1 -> Mux/4
  Divide4/1 -> Product17/1
  Add5/1 -> Mux/3
  Product26/1 -> Add5/2
  Constant7/1 -> Product30/1
  Trigonometric Function/1 -> Divide4/1, Gain1/1, Subsystem9/1(In1), Subsystem7/2(In2), Subsystem6/1(In1), Subsystem2/3(In3), Subsystem5/1(In1), Subsystem4/3(In3)
  Constant14/1 -> Product37/1
  Gain/1 -> Product25/1
  Trigonometric Function5/1 -> Subsystem6/2(In2), Subsystem5/5(In5), Subsystem4/5(In5), Subsystem1/2(In2), Subsystem2/2(In2)
  Subsystem8/1(Out1) -> Product27/1
  Subsystem3/1(Out1) -> Product1/1
  Subsystem6/1(Out1) -> Product3/1
  Demux7/2 -> Product26/2
  Constant20/1 -> Product16/1
  Subsystem7/1(Out1) -> Product26/1
  Demux7/5 -> Product29/2
  Constant15/1 -> Product15/1
  Constant16/1 -> Product14/1
  Demux3/2 -> Product14/2
  Product15/1 -> Add3/3
  Constant17/1 -> Product13/1
  Product14/1 -> Add3/2
  Constant11/1 -> Product7/1
  Trigonometric Function4/1 -> Subsystem6/5(In5), Subsystem2/5(In5), Subsystem3/2(In2), Subsystem5/2(In2), Subsystem4/2(In2)
  Subsystem4/1(Out1) -> Product32/1
  Product13/1 -> Add3/1
  Product16/1 -> Add3/4
  Demux3/1 -> Product13/2
  Demux3/4 -> Product16/2
  Demux3/3 -> Product15/2
  Trigonometric Function2/1 -> Subsystem10/2(In2), Subsystem9/2(In2), Gain/1, Subsystem6/4(In4), Subsystem2/4(In4), Subsystem5/4(In4), Subsystem4/4(In4)
  Constant1/1 -> Product36/1
  Product17/1 -> Add3/5
  Demux5/3 -> Product3/2
  Product6/1 -> Add1/6
  Demux5/5 -> Product5/2
  Demux5/4 -> Product4/2
  Demux5/1 -> Product1/2
  Demux1/1 -> Trigonometric Function/1, Trigonometric Function1/1  "phi"
  Constant4/1 -> Product6/1
  Constant2/1 -> Product34/1
  Constant/1 -> Product35/1
  Demux8/6 -> Product42/2
  Demux3/5 -> Product17/2
  Product4/1 -> Add1/4
  Constant18/1 -> Product40/1
  Product37/1 -> Add7/1
  Demux2/6 -> Product12/2
  Demux8/4 -> Product40/2
  Gain1/1 -> Subsystem11/1(In1)
  Product42/1 -> Add7/6
  Constant3/1 -> Product5/1
  Product8/1 -> Add2/2
  Demux8/5 -> Product41/2
  Product1/1 -> Add1/1
  Demux8/3 -> Product39/2
  Product3/1 -> Add1/3
  Divide2/1 -> Product11/1
  Product18/1 -> Add3/6
  Demux1/3 -> Trigonometric Function5/1, Trigonometric Function4/1  "psi"
  Constant5/1 -> Product4/1
  Demux5/2 -> Product2/2
  Divide/1 -> Product41/1
  Product32/1 -> Add6/2
  Product2/1 -> Add1/2
  Product34/1 -> Add6/4
  Demux6/1 -> Product31/2
  Demux6/6 -> Product36/2
  Product41/1 -> Add7/5
  Demux6/5 -> Product35/2
  Product5/1 -> Add1/5
  Constant9/1 -> Product9/1
  Demux3/6 -> Product18/2
  Product33/1 -> Add6/3
  Demux1/2 -> Trigonometric Function2/1, Trigonometric Function3/1  "theta"
  Demux6/4 -> Product34/2
  Demux6/3 -> Product33/2
  Demux5/6 -> Product6/2
  Product36/1 -> Add6/6
  Demux6/2 -> Product32/2
  Subsystem2/1(Out1) -> Product2/1
  Product40/1 -> Add7/4
  Demux8/1 -> Product37/2
  Product31/1 -> Add6/1
  Product35/1 -> Add6/5
  In2/1 -> Demux1/1

== system Simulink_Control_BlueROVtest6/Observation/RadToAngle ==
  rad : Inport
  Constant6 : Constant  Value=180
  Constant7 : Constant  Value=3.141592657
  Divide1 : Product  Inputs=*/*
  angle : Outport
  wires:
  Constant6/1 -> Divide1/3
  rad/1 -> Divide1/1
  Divide1/1 -> angle/1
  Constant7/1 -> Divide1/2

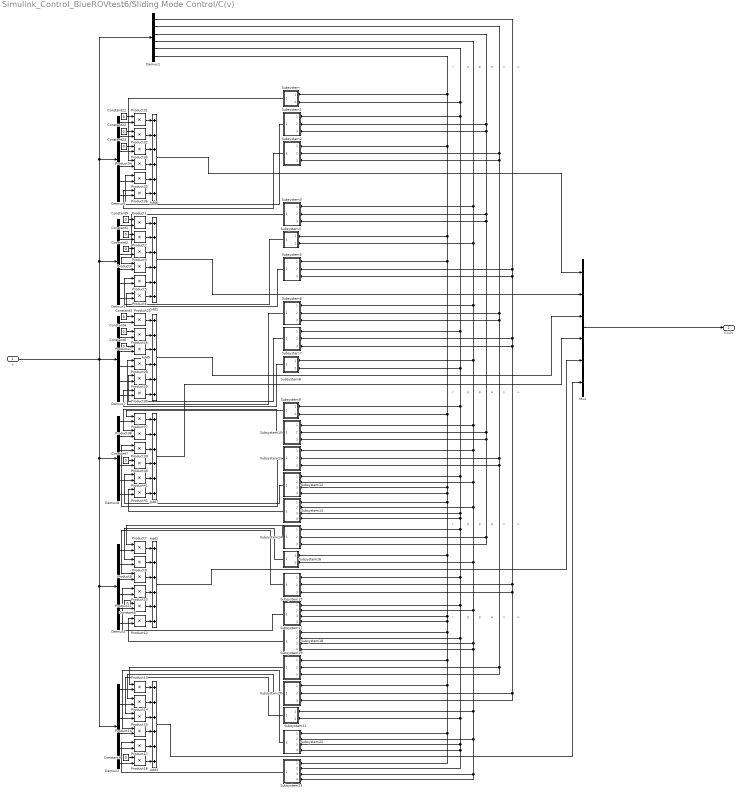
== system Simulink_Control_BlueROVtest6/Sliding Mode Control/C(v) ==
  note: u
  note: v
  note: w
  note: p
  note: q
  note: r
  note: v
  note: p
  note: u
  note: w
  note: q
  note: r
  note: v
  note: r
  note: w
  note: u
  note: q
  note: p
  note: v
  note: r
  note: w
  note: u
  note: q
  note: p
  v : Inport
  Add{1..3,5..7} (6 alike) : Sum  Inputs=++++++
  Constant{1..9,21..23} (12 alike) : Constant  Value=0
  Demux{1..3,5..8} (7 alike) : Demux  Outputs=6
  Mux : Mux  Inputs=6
  Product{1..18,25..42} (36 alike) : Product
  Subsystem : Subsystem
  Subsystem1 : Subsystem
  Subsystem10 : Subsystem
  Subsystem11 : Subsystem
  Subsystem12 : Subsystem
  Subsystem13 : Subsystem
  Subsystem14 : Subsystem
  Subsystem15 : Subsystem
  Subsystem16 : Subsystem
  Subsystem17 : Subsystem
  Subsystem18 : Subsystem
  Subsystem19 : Subsystem
  Subsystem2 : Subsystem
  Subsystem20 : Subsystem
  Subsystem21 : Subsystem
  Subsystem22 : Subsystem
  Subsystem23 : Subsystem
  Subsystem3 : Subsystem
  Subsystem4 : Subsystem
  Subsystem5 : Subsystem
  Subsystem6 : Subsystem
  Subsystem7 : Subsystem
  Subsystem8 : Subsystem
  Subsystem9 : Subsystem
  C(v)v : Outport  VectorParamsAs1DForOutWhenUnconnected=off
  wires:
  v/1 -> Demux5/1, Demux6/1, Demux1/1, Demux7/1, Demux8/1, Demux3/1, Demux2/1
  Product39/1 -> Add7/3
  Demux8/2 -> Product38/2
  Product36/1 -> Add6/6
  Product31/1 -> Add6/1
  Product35/1 -> Add6/5
  Demux6/2 -> Product32/2
  Demux6/4 -> Product34/2
  Demux6/5 -> Product35/2
  Product33/1 -> Add6/3
  Demux6/3 -> Product33/2
  Product5/1 -> Add1/5
  Demux5/2 -> Product2/2
  Product32/1 -> Add6/2
  Product41/1 -> Add7/5
  Product34/1 -> Add6/4
  Product2/1 -> Add1/2
  Demux8/5 -> Product41/2
  Product1/1 -> Add1/1
  Product18/1 -> Add3/6
  Product3/1 -> Add1/3
  Demux8/3 -> Product39/2
  Product8/1 -> Add2/2
  Demux2/6 -> Product12/2
  Product4/1 -> Add1/4
  Product37/1 -> Add7/1
  Demux5/1 -> Product1/2
  Demux8/6 -> Product42/2
  Demux5/4 -> Product4/2
  Demux5/5 -> Product5/2
  Product17/1 -> Add3/5
  Demux5/3 -> Product3/2
  Demux6/1 -> Product31/2
  Product13/1 -> Add3/1
  Product14/1 -> Add3/2
  Product40/1 -> Add7/4
  Product15/1 -> Add3/3
  Demux8/4 -> Product40/2
  Demux7/2 -> Product26/2
  Product42/1 -> Add7/6
  Product12/1 -> Add2/6
  Product26/1 -> Add5/2
  Product6/1 -> Add1/6
  Demux6/6 -> Product36/2
  Demux5/6 -> Product6/2
  Product29/1 -> Add5/5
  Product28/1 -> Add5/4
  Demux7/3 -> Product27/2
  Product16/1 -> Add3/4
  Product10/1 -> Add2/4
  Demux7/5 -> Product29/2
  Product9/1 -> Add2/3
  Product38/1 -> Add7/2
  Demux2/4 -> Product10/2
  Demux2/2 -> Product8/2
  Demux8/1 -> Product37/2
  Demux2/5 -> Product11/2
  Product7/1 -> Add2/1
  Product11/1 -> Add2/5
  Mux/1 -> C(v)v/1
  Demux7/4 -> Product28/2
  Demux2/1 -> Product7/2
  Demux7/6 -> Product30/2
  Product25/1 -> Add5/1
  Product27/1 -> Add5/3
  Product30/1 -> Add5/6
  Demux7/1 -> Product25/2
  Demux2/3 -> Product9/2
  Constant21/1 -> Product31/1
  Constant22/1 -> Product32/1
  Constant23/1 -> Product33/1
  Demux3/6 -> Product18/2
  Demux3/5 -> Product17/2
  Demux3/4 -> Product16/2
  Demux3/3 -> Product15/2
  Demux3/2 -> Product14/2
  Demux3/1 -> Product13/2
  Constant5/1 -> Product1/1
  Constant1/1 -> Product2/1
  Constant2/1 -> Product3/1
  Constant3/1 -> Product25/1
  Constant4/1 -> Product26/1
  Constant6/1 -> Product27/1
  Constant7/1 -> Product40/1
  Constant8/1 -> Product11/1
  Constant9/1 -> Product18/1
  Demux1/1 -> Subsystem5/2(In2), Subsystem15/2(In2), Subsystem15/3(In3), Subsystem20/2(In2), Subsystem20/3(In3), Subsystem7/3(In3), Subsystem7/2(In2), Subsystem5/3(In3)
  Demux1/2 -> Subsystem11/3(In3), Subsystem19/2(In2), Subsystem19/3(In3), Subsystem11/2(In2), Subsystem6/3(In3), Subsystem6/2(In2), Subsystem2/3(In3), Subsystem2/2(In2)
  Demux1/3 -> Subsystem3/2(In2), Subsystem3/3(In3), Subsystem10/2(In2), Subsystem10/3(In3), Subsystem14/2(In2), Subsystem14/3(In3), Subsystem1/3(In3), Subsystem1/2(In2)
  Subsystem/1(Out1) -> Product34/1
  Subsystem1/1(Out1) -> Product35/1
  Subsystem2/1(Out1) -> Product36/1
  Add6/1 -> Mux/1
  Subsystem3/1(Out1) -> Product4/1
  Subsystem4/1(Out1) -> Product5/1
  Subsystem5/1(Out1) -> Product6/1
  Add1/1 -> Mux/2
  Subsystem6/1(Out1) -> Product28/1
  Subsystem7/1(Out1) -> Product29/1
  Subsystem8/1(Out1) -> Product30/1
  Add5/1 -> Mux/3
  Subsystem9/1(Out1) -> Product37/1
  Subsystem10/1(Out1) -> Product38/1
  Subsystem11/1(Out1) -> Product39/1
  Subsystem12/1(Out1) -> Product41/1
  Subsystem13/1(Out1) -> Product42/1
  Add7/1 -> Mux/4
  Subsystem14/1(Out1) -> Product7/1
  Demux1/4 -> Subsystem3/1(In1), Subsystem4/2(In2), Subsystem8/1(In1), Subsystem10/1(In1), Subsystem11/1(In1), Subsystem12/2(In2), Subsystem13/2(In2), Subsystem16/2(In2), Subsystem17/2(In2), Subsystem18/3(In3), Subsystem18/4(In4), Subsystem21/1(In1), Subsystem22/2(In2), Subsystem23/3(In3), Subsystem23/4(In4), Subsystem6/1(In1)
  Subsystem16/1(Out1) -> Product8/1
  Subsystem15/1(Out1) -> Product9/1
  Demux1/6 -> Subsystem4/1(In1), Subsystem5/1(In1), Subsystem12/4(In4), Subsystem13/1(In1), Subsystem16/1(In1), Subsystem17/4(In4), Subsystem18/1(In1), Subsystem19/1(In1), Subsystem20/1(In1), Subsystem22/1(In1), Subsystem23/1(In1), Subsystem17/3(In3), Subsystem12/3(In3), Subsystem9/2(In2), Subsystem2/1(In1), Subsystem/1(In1)
  Subsystem17/1(Out1) -> Product10/1
  Subsystem18/1(Out1) -> Product12/1
  Subsystem19/1(Out1) -> Product13/1
  Add2/1 -> Mux/5
  Subsystem20/1(Out1) -> Product14/1
  Subsystem21/1(Out1) -> Product15/1
  Demux1/5 -> Subsystem12/1(In1), Subsystem13/3(In3), Subsystem13/4(In4), Subsystem15/1(In1), Subsystem17/1(In1), Subsystem18/2(In2), Subsystem21/2(In2), Subsystem22/4(In4), Subsystem23/2(In2), Subsystem22/3(In3), Subsystem14/1(In1), Subsystem9/1(In1), Subsystem8/2(In2), Subsystem7/1(In1), Subsystem1/1(In1), Subsystem/2(In2)
  Subsystem22/1(Out1) -> Product16/1
  Subsystem23/1(Out1) -> Product17/1
  Add3/1 -> Mux/6

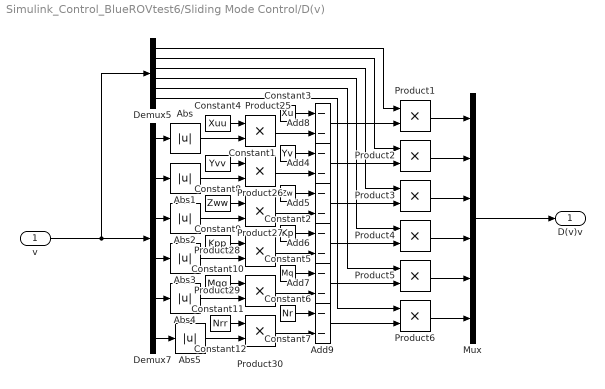
== system Simulink_Control_BlueROVtest6/Sliding Mode Control/D(v) ==
  v : Inport
  Abs{,1..5} (6 alike) : Abs  SaturateOnIntegerOverflow=off
  Add{4..9} (6 alike) : Sum  Inputs=--
  Constant1 : Constant  Value=Yv
  Constant10 : Constant  Value=Kpp
  Constant11 : Constant  Value=Mqq
  Constant12 : Constant  Value=Nrr
  Constant2 : Constant  Value=Zw
  Constant3 : Constant  Value=Xu
  Constant4 : Constant  Value=Xuu
  Constant5 : Constant  Value=Kp
  Constant6 : Constant  Value=Mq
  Constant7 : Constant  Value=Nr
  Constant8 : Constant  Value=Yvv
  Constant9 : Constant  Value=Zww
  Demux5 : Demux  Outputs=6
  Demux7 : Demux  Outputs=6
  Mux : Mux  Inputs=6
  Product{1..6,25..30} (12 alike) : Product
  D(v)v : Outport
  wires:
  Demux7/1 -> Abs/1
  Constant2/1 -> Add5/1
  Demux7/2 -> Abs1/1
  Product2/1 -> Mux/2
  Demux7/6 -> Abs5/1
  Add9/1 -> Product6/2
  Abs2/1 -> Product27/2
  Product27/1 -> Add5/2
  Demux7/3 -> Abs2/1
  v/1 -> Demux5/1, Demux7/1
  Product26/1 -> Add4/2
  Product25/1 -> Add8/2
  Constant9/1 -> Product27/1
  Add7/1 -> Product5/2
  Product29/1 -> Add7/2
  Constant1/1 -> Add4/1
  Add8/1 -> Product1/2
  Constant4/1 -> Product25/1
  Demux5/3 -> Product3/1
  Abs/1 -> Product25/2
  Add5/1 -> Product3/2
  Add4/1 -> Product2/2
  Constant11/1 -> Product29/1
  Product3/1 -> Mux/3
  Constant10/1 -> Product28/1
  Abs4/1 -> Product29/2
  Demux7/5 -> Abs4/1
  Demux5/1 -> Product1/1
  Demux7/4 -> Abs3/1
  Constant6/1 -> Add7/1
  Product28/1 -> Add6/2
  Product6/1 -> Mux/6
  Constant3/1 -> Add8/1
  Constant8/1 -> Product26/1
  Demux5/5 -> Product5/1
  Product1/1 -> Mux/1
  Demux5/6 -> Product6/1
  Product5/1 -> Mux/5
  Constant12/1 -> Product30/1
  Constant5/1 -> Add6/1
  Abs1/1 -> Product26/2
  Abs5/1 -> Product30/2
  Constant7/1 -> Add9/1
  Add6/1 -> Product4/2
  Demux5/4 -> Product4/1
  Abs3/1 -> Product28/2
  Product4/1 -> Mux/4
  Product30/1 -> Add9/2
  Demux5/2 -> Product2/1
  Mux/1 -> D(v)v/1

== system Simulink_Control_BlueROVtest6/Sliding Mode Control/de ==
  In1 : Inport
  Demux : Demux  Outputs=6
  To Workspace : ToWorkspace  VariableName=de_X  SampleTime=-1
  To Workspace1 : ToWorkspace  VariableName=de_Y  SampleTime=-1
  To Workspace2 : ToWorkspace  VariableName=de_Z  SampleTime=-1
  wires:
  In1/1 -> Demux/1
  Demux/1 -> To Workspace/1
  Demux/2 -> To Workspace1/1
  Demux/3 -> To Workspace2/1

== system Simulink_Control_BlueROVtest6/Sliding Mode Control/e ==
  In1 : Inport
  Demux : Demux  Outputs=6
  To Workspace : ToWorkspace  VariableName=e_X  SampleTime=-1
  To Workspace1 : ToWorkspace  VariableName=e_Y  SampleTime=-1
  To Workspace2 : ToWorkspace  VariableName=e_Z  SampleTime=-1
  wires:
  In1/1 -> Demux/1
  Demux/1 -> To Workspace/1
  Demux/2 -> To Workspace1/1
  Demux/3 -> To Workspace2/1

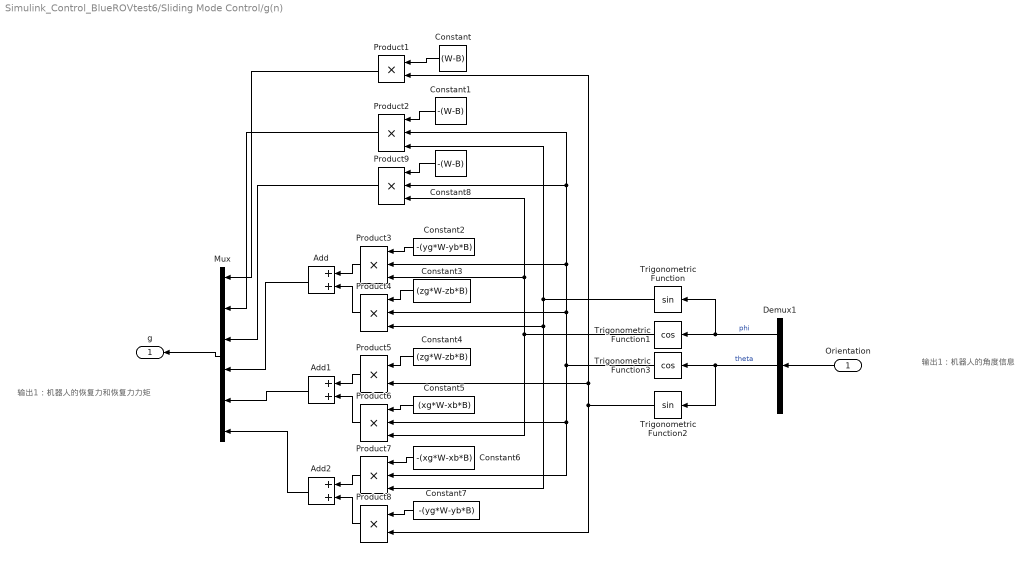
== system Simulink_Control_BlueROVtest6/Sliding Mode Control/g(n) ==
  note: 输出1：机器人的恢复力和恢复力力矩
  note: 输出1：机器人的角度信息
  Orientation : Inport
  Add : Sum
  Add1 : Sum
  Add2 : Sum
  Constant : Constant  Value=(W-B)
  Constant1 : Constant  Value=-(W-B)
  Constant2 : Constant  Value=-(yg*W-yb*B)
  Constant3 : Constant  Value=(zg*W-zb*B)
  Constant4 : Constant  Value=(zg*W-zb*B)
  Constant5 : Constant  Value=(xg*W-xb*B)
  Constant6 : Constant  Value=-(xg*W-xb*B)
  Constant7 : Constant  Value=-(yg*W-yb*B)
  Constant8 : Constant  Value=-(W-B)
  Demux1 : Demux  Outputs=3
  Mux : Mux  Inputs=6
  Product1 : Product
  Product{2..4,6..7,9} (6 alike) : Product  Inputs=3
  Product5 : Product
  Product8 : Product
  Trigonometric Function : Trigonometry
  Trigonometric Function1 : Trigonometry  Operator=cos
  Trigonometric Function2 : Trigonometry
  Trigonometric Function3 : Trigonometry  Operator=cos
  g : Outport  VectorParamsAs1DForOutWhenUnconnected=off
  wires:
  Demux1/1 -> Trigonometric Function/1, Trigonometric Function1/1  "phi"
  Demux1/2 -> Trigonometric Function2/1, Trigonometric Function3/1  "theta"
  Orientation/1 -> Demux1/1
  Mux/1 -> g/1
  Product1/1 -> Mux/1
  Constant/1 -> Product1/1
  Trigonometric Function2/1 -> Product1/2, Product5/2, Product8/2
  Constant1/1 -> Product2/1
  Trigonometric Function/1 -> Product2/3, Product7/3, Product4/3
  Product2/1 -> Mux/2
  Product7/1 -> Add2/1
  Product8/1 -> Add2/2
  Product6/1 -> Add1/2
  Constant5/1 -> Product6/1
  Constant2/1 -> Product3/1
  Constant4/1 -> Product5/1
  Product4/1 -> Add/2
  Constant3/1 -> Product4/1
  Product3/1 -> Add/1
  Product5/1 -> Add1/1
  Constant7/1 -> Product8/1
  Constant8/1 -> Product9/1
  Product9/1 -> Mux/3
  Add/1 -> Mux/4
  Add1/1 -> Mux/5
  Constant6/1 -> Product7/1
  Add2/1 -> Mux/6
  Trigonometric Function1/1 -> Product3/3, Product9/3, Product6/3
  Trigonometric Function3/1 -> Product4/2, Product3/2, Product9/2, Product2/2, Product7/2, Product6/2

== system Simulink_Control_BlueROVtest6/Subsystem1/AngleToRad ==
  Angle : Inport
  Constant1 : Constant  Value=180
  Constant2 : Constant  Value=3.141592657
  Divide3 : Product  Inputs=*/*
  Rad : Outport
  wires:
  Divide3/1 -> Rad/1
  Constant2/1 -> Divide3/3
  Constant1/1 -> Divide3/2
  Angle/1 -> Divide3/1

== system Simulink_Control_BlueROVtest6/BlueRov2Heavy/C(v)/Subsystem ==
  In1 : Inport
  In2 : Inport  Port=2
  Add4 : Sum
  Constant : Constant  Value=zg
  Constant10 : Constant  Value=yg
  Gain : Gain  Gain=m
  Product19 : Product
  Product20 : Product
  Out1 : Outport  VectorParamsAs1DForOutWhenUnconnected=off
  wires:
  Product20/1 -> Add4/2
  Product19/1 -> Add4/1
  In1/1 -> Product19/2
  Constant/1 -> Product19/1
  Gain/1 -> Out1/1
  Constant10/1 -> Product20/1
  Add4/1 -> Gain/1
  In2/1 -> Product20/2

== system Simulink_Control_BlueROVtest6/BlueRov2Heavy/C(v)/Subsystem1 ==
  In1 : Inport
  In2 : Inport  Port=2
  In3 : Inport  Port=3
  Add4 : Sum  Inputs=+-
  Add8 : Sum  Inputs=-+
  Constant : Constant  Value=xg
  Constant10 : Constant
  Constant11 : Constant  Value=-Zwdot
  Gain : Gain  Gain=m
  Product19 : Product
  Product20 : Product
  Product21 : Product
  Out1 : Outport  VectorParamsAs1DForOutWhenUnconnected=off
  wires:
  Product20/1 -> Add4/2
  Constant11/1 -> Product21/1
  Gain/1 -> Add8/1
  Product19/1 -> Add4/1
  Constant/1 -> Product19/1
  Product21/1 -> Add8/2
  Add4/1 -> Gain/1
  Constant10/1 -> Product20/1
  Add8/1 -> Out1/1
  In1/1 -> Product19/2
  In3/1 -> Product21/2
  In2/1 -> Product20/2

== system Simulink_Control_BlueROVtest6/BlueRov2Heavy/C(v)/Subsystem10 ==
  In1 : Inport
  In2 : Inport  Port=2
  In3 : Inport  Port=3
  Add4 : Sum
  Add8 : Sum
  Constant : Constant  Value=yg
  Constant10 : Constant
  Constant11 : Constant  Value=-Zwdot
  Gain : Gain  Gain=m
  Product19 : Product
  Product20 : Product
  Product21 : Product
  Out1 : Outport  VectorParamsAs1DForOutWhenUnconnected=off
  wires:
  In2/1 -> Product20/2
  In3/1 -> Product21/2
  In1/1 -> Product19/2
  Add8/1 -> Out1/1
  Constant10/1 -> Product20/1
  Add4/1 -> Gain/1
  Product21/1 -> Add8/2
  Constant/1 -> Product19/1
  Product19/1 -> Add4/1
  Gain/1 -> Add8/1
  Constant11/1 -> Product21/1
  Product20/1 -> Add4/2

== system Simulink_Control_BlueROVtest6/BlueRov2Heavy/C(v)/Subsystem11 ==
  In1 : Inport
  In2 : Inport  Port=2
  In3 : Inport  Port=3
  Add4 : Sum  Inputs=+-
  Add8 : Sum
  Constant : Constant  Value=zg
  Constant10 : Constant
  Constant11 : Constant  Value=Yvdot
  Gain : Gain  Gain=m
  Product19 : Product
  Product20 : Product
  Product21 : Product
  Out1 : Outport  VectorParamsAs1DForOutWhenUnconnected=off
  wires:
  Product20/1 -> Add4/2
  Constant11/1 -> Product21/1
  Gain/1 -> Add8/1
  Product19/1 -> Add4/1
  Constant/1 -> Product19/1
  Product21/1 -> Add8/2
  Add4/1 -> Gain/1
  Constant10/1 -> Product20/1
  Add8/1 -> Out1/1
  In1/1 -> Product19/2
  In3/1 -> Product21/2
  In2/1 -> Product20/2

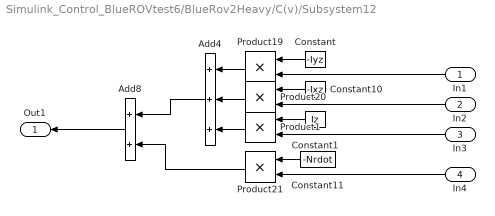
== system Simulink_Control_BlueROVtest6/BlueRov2Heavy/C(v)/Subsystem12 ==
  In1 : Inport
  In2 : Inport  Port=2
  In3 : Inport  Port=3
  In4 : Inport  Port=4
  Add4 : Sum  Inputs=+++
  Add8 : Sum
  Constant : Constant  Value=-Iyz
  Constant1 : Constant  Value=Iz
  Constant10 : Constant  Value=-Ixz
  Constant11 : Constant  Value=-Nrdot
  Product{1,19..21} (4 alike) : Product
  Out1 : Outport  VectorParamsAs1DForOutWhenUnconnected=off
  wires:
  In2/1 -> Product20/2
  In1/1 -> Product19/2
  Add8/1 -> Out1/1
  Constant10/1 -> Product20/1
  Product21/1 -> Add8/2
  Constant/1 -> Product19/1
  Product19/1 -> Add4/1
  Add4/1 -> Add8/1
  Constant11/1 -> Product21/1
  Product20/1 -> Add4/2
  Product1/1 -> Add4/3
  Constant1/1 -> Product1/1
  In4/1 -> Product21/2
  In3/1 -> Product1/2
